simulink model "matrix_rdwr_transpose_fpga"  (R2020b)
settings: Solver=FixedStepDiscrete  StartTime=0.0  StopTime=inf  RelTol=1e-3
InitFcn:
  | %hsb_FFT_2D_init;
values from neighbouring files (symbols this model uses):
  N1 = 20    [matrix_init.m]
  N2 = 20    [matrix_init.m]
libraries: hwlogicconnlib x4, simulink x1, hdlsllib x1
settings Model: DataTypeOverride=Off  Creator=The MathWorks, Inc.  LastModifiedBy=darenlee
settings DataIOCC: LimitDataPoints=on  SaveFormat=Array  SaveOutput=off  SaveTime=off  ReturnWorkspaceOutputs=off
settings OptimizationCC: BlockReduction=off  ConditionallyExecuteInputs=off  DefaultParameterBehavior=Inlined  LifeSpan=inf
settings DebuggingCC: AlgebraicLoopMsg=error  SolverPrmCheckMsg=warning  InheritedTsInSrcMsg=none  SingleTaskRateTransMsg=error  IntegerOverflowMsg=none  ParameterPrecisionLossMsg=none  AllowSymbolicDim=off  SFUnexpectedBacktrackingDiag=warning  SFNoUnconditionalDefaultTransitionDiag=warning  SFExecutionAtInitializationDiag=none  IntegerSaturationMsg=none  ArithmeticOperatorsInVariantConditions=warning
settings HardwareCC: ProdBitPerPointer=32  ProdBitPerSizeT=32  ProdBitPerPtrDiffT=32  ProdLargestAtomicFloat=None  ProdIntDivRoundTo=Undefined  ProdEndianess=Unspecified  ProdWordSize=32  ProdHWDeviceType=ASIC/FPGA->ASIC/FPGA  TargetBitPerPointer=64  TargetBitPerSizeT=64  TargetBitPerPtrDiffT=64  TargetLongLongMode=on  TargetIntDivRoundTo=Zero  TargetEndianess=LittleEndian  TargetWordSize=64  TargetHWDeviceType=Custom Processor->MATLAB Host Computer  ProdEqTarget=off
settings ModelReferenceCC: PropagateSignalLabelsOutOfModel=off
settings SFSimCC: SimUseLocalCustomCode=off  CustomCodeUndefinedFunction=UseInterfaceOnly
settings RTWCC: RTWUseLocalCustomCode=off
settings CodeAppCC: StateflowObjectComments=on
settings GRTTargetCC: TargetLangStandard=C89/C90 (ANSI)
settings ConfigComp: CovMetricSettings=dw  CovSaveCumulativeToWorkspaceVar=on  CovSaveSingleToWorkspaceVar=on  CovExternalEMLEnable=off  CovSFcnEnable=off
settings SimscapeCC: SimscapeNormalizeSystem=off

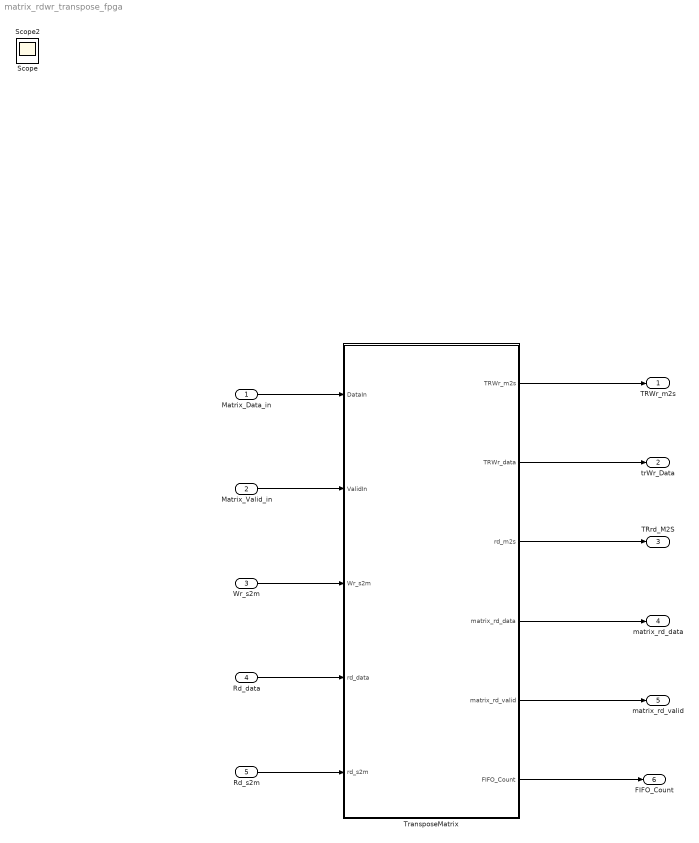
== system matrix_rdwr_transpose_fpga ==
  Matrix_Data_in : Inport  OutDataTypeStr=uint32
  Matrix_Valid_in : Inport  Port=2  OutDataTypeStr=boolean
  Wr_s2m : Inport  Port=3  OutDataTypeStr=Bus: WriteControlS2MBusObj  PortDimensions=1  BusOutputAsStruct=on
  Rd_data : Inport  Port=4  OutDataTypeStr=fixdt(0,32,0)  PortDimensions=1
  Rd_s2m : Inport  Port=5  OutDataTypeStr=Bus: ReadControlS2MBusObj  BusOutputAsStruct=on
  TransposeMatrix : Subsystem  TreatAsAtomicUnit=on
  TRWr_m2s : Outport  OutDataTypeStr=Bus: WriteControlM2SBusObj  PortDimensions=1  VectorParamsAs1DForOutWhenUnconnected=off  BusOutputAsStruct=on
  trWr_Data : Outport  Port=2  PortDimensions=1  VectorParamsAs1DForOutWhenUnconnected=off  BusOutputAsStruct=on
  TRrd_M2S : Outport  Port=3  OutDataTypeStr=Bus: ReadControlM2SBusObj  BusOutputAsStruct=on
  matrix_rd_data : Outport  Port=4
  matrix_rd_valid : Outport  Port=5
  FIFO_Count : Outport  Port=6
  Scope : Scope
  Scope2 : Scope
  wires:
  Rd_data/1 -> TransposeMatrix/4(rd_data)
  TransposeMatrix/5(matrix_rd_valid) -> matrix_rd_valid/1
  Matrix_Valid_in/1 -> TransposeMatrix/2(ValidIn)
  TransposeMatrix/4(matrix_rd_data) -> matrix_rd_data/1
  Rd_s2m/1 -> TransposeMatrix/5(rd_s2m)
  Matrix_Data_in/1 -> TransposeMatrix/1(DataIn)
  TransposeMatrix/2(TRWr_data) -> trWr_Data/1
  Wr_s2m/1 -> TransposeMatrix/3(Wr_s2m)
  TransposeMatrix/3(rd_m2s) -> TRrd_M2S/1
  TransposeMatrix/1(TRWr_m2s) -> TRWr_m2s/1
  TransposeMatrix/6(FIFO_Count) -> FIFO_Count/1

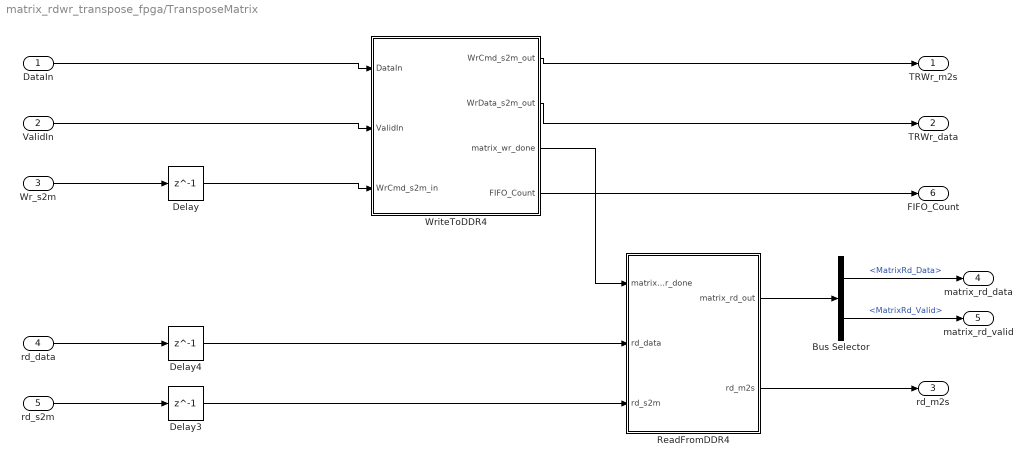
== system matrix_rdwr_transpose_fpga/TransposeMatrix ==
  DataIn : Inport
  ValidIn : Inport  Port=2
  Wr_s2m : Inport  Port=3  SampleTime=1
  rd_data : Inport  Port=4  SampleTime=1
  rd_s2m : Inport  Port=5  SampleTime=1
  Bus Selector : BusSelector  OutputSignals=MatrixRd_Data,MatrixRd_Valid
  Delay : Delay  DelayLength=1
  Delay3 : Delay  DelayLength=1
  Delay4 : Delay  DelayLength=1
  ReadFromDDR4 : Subsystem
  WriteToDDR4 : Subsystem
  TRWr_m2s : Outport  SampleTime=1  VectorParamsAs1DForOutWhenUnconnected=off
  TRWr_data : Outport  Port=2  SampleTime=1  VectorParamsAs1DForOutWhenUnconnected=off
  rd_m2s : Outport  Port=3
  matrix_rd_data : Outport  Port=4
  matrix_rd_valid : Outport  Port=5
  FIFO_Count : Outport  Port=6
  wires:
  rd_data/1 -> Delay4/1
  rd_s2m/1 -> Delay3/1
  Wr_s2m/1 -> Delay/1
  DataIn/1 -> WriteToDDR4/1(DataIn)
  ValidIn/1 -> WriteToDDR4/2(ValidIn)
  Delay/1 -> WriteToDDR4/3(WrCmd_s2m_in)
  WriteToDDR4/1(WrCmd_s2m_out) -> TRWr_m2s/1
  WriteToDDR4/2(WrData_s2m_out) -> TRWr_data/1
  Delay4/1 -> ReadFromDDR4/2(rd_data)
  Delay3/1 -> ReadFromDDR4/3(rd_s2m)
  ReadFromDDR4/2(rd_m2s) -> rd_m2s/1
  WriteToDDR4/3(matrix_wr_done) -> ReadFromDDR4/1(matrix_wr_done)
  ReadFromDDR4/1(matrix_rd_out) -> Bus Selector/1
  Bus Selector/1 -> matrix_rd_data/1  "<MatrixRd_Data>"
  Bus Selector/2 -> matrix_rd_valid/1  "<MatrixRd_Valid>"
  WriteToDDR4/4(FIFO_Count) -> FIFO_Count/1

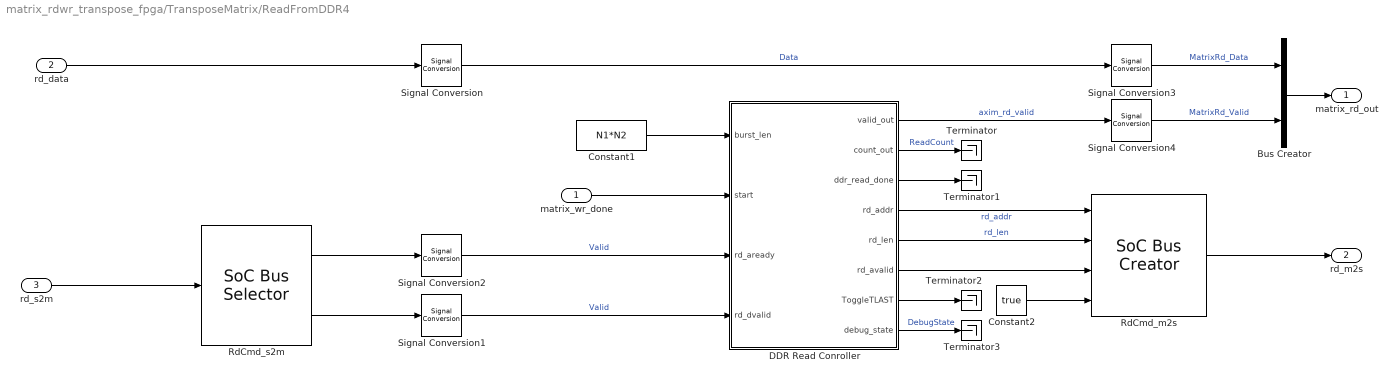
== system matrix_rdwr_transpose_fpga/TransposeMatrix/ReadFromDDR4 ==
  matrix_wr_done : Inport
  rd_data : Inport  Port=2
  rd_s2m : Inport  Port=3
  Bus Creator : BusCreator  Inputs=2
  Constant1 : Constant  Value=N1*N2  OutDataTypeStr=uint32  SampleTime=-1
  Constant2 : Constant  Value=true  SampleTime=-1
  DDR Read Conroller : MATLAB Function  TreatAsAtomicUnit=on
  RdCmd_m2s : hwlogicconnlib/SoC Bus Creator  Protocol=Random access read  ctrltype=Ready
      settings: SourceProductBaseCode=HW
  "RdCmd_s2m " : hwlogicconnlib/SoC Bus Selector  Protocol=Random access read  ctrltype=Valid
      settings: SourceProductBaseCode=HW
  Signal Conversion{,1..4} (5 alike) : SignalConversion  OverrideOpt=off
  Terminator{,1..3} (4 alike) : Terminator
  matrix_rd_out : Outport
  rd_m2s : Outport  Port=2
  wires:
  Signal Conversion1/1 -> DDR Read Conroller/4(rd_dvalid)  "Valid"
  "RdCmd_s2m "/2 -> Signal Conversion1/1
  Signal Conversion/1 -> Signal Conversion3/1  "Data"
  DDR Read Conroller/5(rd_len) -> RdCmd_m2s/2  "rd_len"
  RdCmd_m2s/1 -> rd_m2s/1
  rd_data/1 -> Signal Conversion/1
  rd_s2m/1 -> "RdCmd_s2m "/1
  matrix_wr_done/1 -> DDR Read Conroller/2(start)
  Constant1/1 -> DDR Read Conroller/1(burst_len)
  "RdCmd_s2m "/1 -> Signal Conversion2/1
  Signal Conversion2/1 -> DDR Read Conroller/3(rd_aready)  "Valid"
  DDR Read Conroller/2(count_out) -> Terminator/1  "ReadCount"
  DDR Read Conroller/1(valid_out) -> Signal Conversion4/1  "axim_rd_valid"
  DDR Read Conroller/3(ddr_read_done) -> Terminator1/1
  DDR Read Conroller/4(rd_addr) -> RdCmd_m2s/1  "rd_addr"
  DDR Read Conroller/6(rd_avalid) -> RdCmd_m2s/3
  Constant2/1 -> RdCmd_m2s/4
  DDR Read Conroller/7(ToggleTLAST) -> Terminator2/1
  DDR Read Conroller/8(debug_state) -> Terminator3/1  "DebugState"
  Signal Conversion3/1 -> Bus Creator/1  "MatrixRd_Data"
  Signal Conversion4/1 -> Bus Creator/2  "MatrixRd_Valid"
  Bus Creator/1 -> matrix_rd_out/1

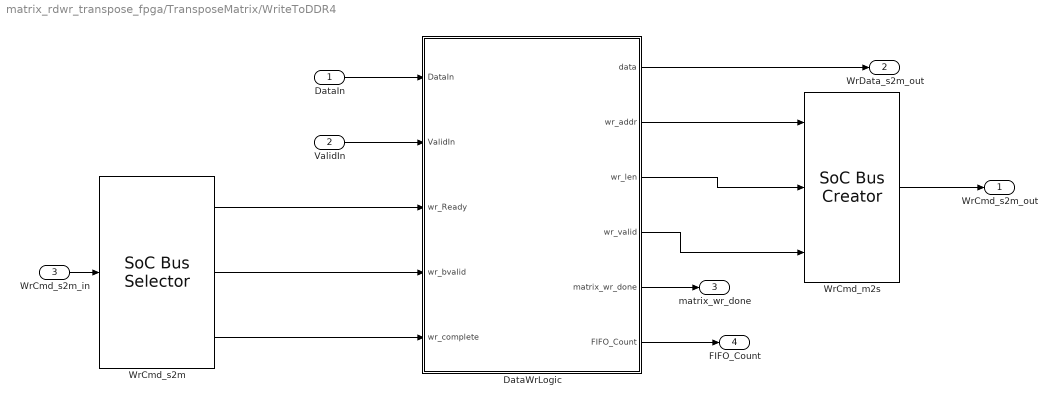
== system matrix_rdwr_transpose_fpga/TransposeMatrix/WriteToDDR4 ==
  DataIn : Inport
  ValidIn : Inport  Port=2
  WrCmd_s2m_in : Inport  Port=3
  DataWrLogic : Subsystem
  WrCmd_m2s : hwlogicconnlib/SoC Bus Creator  Protocol=Random access write  ctrltype=Valid
      settings: SourceProductBaseCode=HW
  WrCmd_s2m : hwlogicconnlib/SoC Bus Selector  Protocol=Random access write  ctrltype=Ready
      settings: SourceProductBaseCode=HW
  WrCmd_s2m_out : Outport
  WrData_s2m_out : Outport  Port=2
  matrix_wr_done : Outport  Port=3
  FIFO_Count : Outport  Port=4
  wires:
  DataWrLogic/4(wr_valid) -> WrCmd_m2s/3
  DataWrLogic/3(wr_len) -> WrCmd_m2s/2
  ValidIn/1 -> DataWrLogic/2(ValidIn)
  DataWrLogic/2(wr_addr) -> WrCmd_m2s/1
  DataWrLogic/1(data) -> WrData_s2m_out/1
  WrCmd_s2m/3 -> DataWrLogic/5(wr_complete)
  WrCmd_s2m/2 -> DataWrLogic/4(wr_bvalid)
  DataIn/1 -> DataWrLogic/1(DataIn)
  WrCmd_m2s/1 -> WrCmd_s2m_out/1
  WrCmd_s2m/1 -> DataWrLogic/3(wr_Ready)
  WrCmd_s2m_in/1 -> WrCmd_s2m/1
  DataWrLogic/5(matrix_wr_done) -> matrix_wr_done/1
  DataWrLogic/6(FIFO_Count) -> FIFO_Count/1

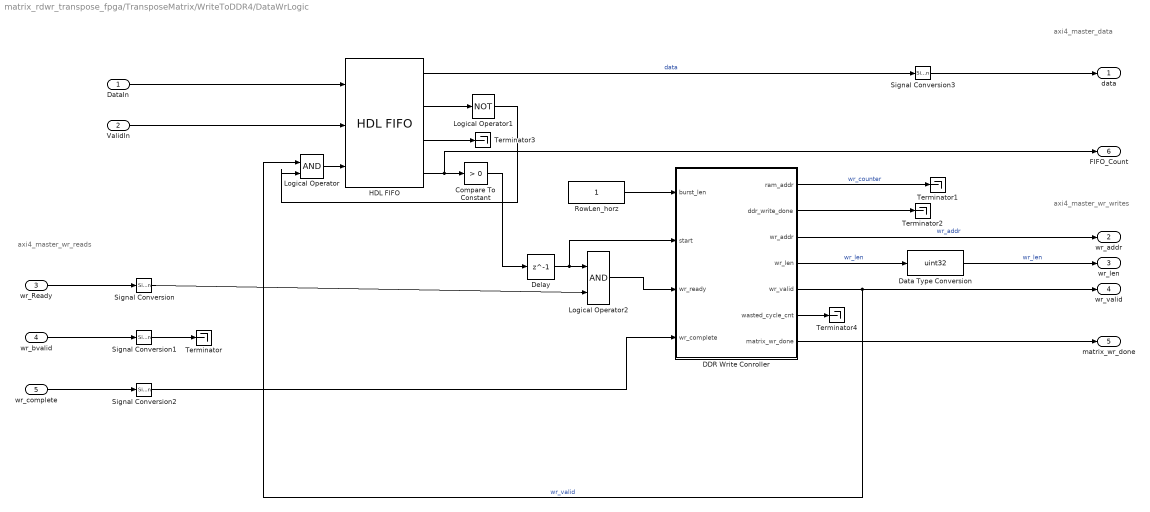
== system matrix_rdwr_transpose_fpga/TransposeMatrix/WriteToDDR4/DataWrLogic ==
  note: axi4_master_wr_reads
  note: axi4_master_wr_writes
  note: axi4_master_data
  DataIn : Inport
  ValidIn : Inport  Port=2
  wr_Ready : Inport  Port=3
  wr_bvalid : Inport  Port=4
  wr_complete : Inport  Port=5
  Compare To Constant : simulink/Logic and Bit Operations/Compare To Constant  relop=>  const=0  OutDataTypeStr=boolean
  DDR Write Conroller : MATLAB Function  TreatAsAtomicUnit=on
  Data Type Conversion : DataTypeConversion  OutDataTypeStr=uint32
  Delay : Delay  DelayLength=1
  HDL FIFO : hdlsllib/HDL RAMs/HDL FIFO  fifo_size=8192  mode=FWFT  ratio=1  push_msg=Warning  pop_msg=Warning  show_empty=on  show_full=on  show_num=on  LabelModeActiveChoice_Mode=FWFT
      settings: SourceProductBaseCode=SL
  Logical Operator : Logic  IconShape=distinctive  AllPortsSameDT=off  OutDataTypeStr=boolean
  Logical Operator1 : Logic  Operator=NOT  IconShape=distinctive  AllPortsSameDT=off  OutDataTypeStr=boolean
  Logical Operator2 : Logic  IconShape=distinctive  AllPortsSameDT=off  OutDataTypeStr=boolean
  RowLen_horz : Constant  OutDataTypeStr=uint32  SampleTime=-1
  Signal Conversion{,1..3} (4 alike) : SignalConversion  OverrideOpt=off
  Terminator{,1..4} (5 alike) : Terminator
  data : Outport
  wr_addr : Outport  Port=2
  wr_len : Outport  Port=3
  wr_valid : Outport  Port=4
  matrix_wr_done : Outport  Port=5
  FIFO_Count : Outport  Port=6
  wires:
  ValidIn/1 -> HDL FIFO/2
  DDR Write Conroller/4(wr_len) -> Data Type Conversion/1  "wr_len"
  wr_bvalid/1 -> Signal Conversion1/1
  DDR Write Conroller/3(wr_addr) -> wr_addr/1  "wr_addr"
  Data Type Conversion/1 -> wr_len/1  "wr_len"
  DataIn/1 -> HDL FIFO/1
  HDL FIFO/1 -> Signal Conversion3/1  "data"
  wr_complete/1 -> Signal Conversion2/1
  wr_Ready/1 -> Signal Conversion/1
  HDL FIFO/2 -> Logical Operator1/1
  Logical Operator/1 -> HDL FIFO/3
  Signal Conversion/1 -> Logical Operator2/2
  Logical Operator2/1 -> DDR Write Conroller/3(wr_ready)
  Logical Operator1/1 -> Logical Operator/2
  HDL FIFO/4 -> FIFO_Count/1, Compare To Constant/1
  Compare To Constant/1 -> Delay/1
  Signal Conversion2/1 -> DDR Write Conroller/4(wr_complete)
  RowLen_horz/1 -> DDR Write Conroller/1(burst_len)
  Signal Conversion1/1 -> Terminator/1
  DDR Write Conroller/5(wr_valid) -> Logical Operator/1, wr_valid/1  "wr_valid"
  DDR Write Conroller/1(ram_addr) -> Terminator1/1  "wr_counter"
  DDR Write Conroller/2(ddr_write_done) -> Terminator2/1
  Signal Conversion3/1 -> data/1
  HDL FIFO/3 -> Terminator3/1
  Delay/1 -> DDR Write Conroller/2(start), Logical Operator2/1
  DDR Write Conroller/6(wasted_cycle_cnt) -> Terminator4/1
  DDR Write Conroller/7(matrix_wr_done) -> matrix_wr_done/1

== matlab function matrix_rdwr_transpose_fpga/TransposeMatrix/WriteToDDR4/DataWrLogic/DDR Write Conroller ==
  data: ram_addr output; ddr_write_done output; burst_len input; start input boolean; wr_ready input; wr_addr output; wr_len output; wr_valid output; wr_complete input; wasted_cycle_cnt output; matrix_wr_done output; N1 parameter uint32; N2 parameter uint32
function [ram_addr, ddr_write_done, wr_addr, wr_len, wr_valid, wasted_cycle_cnt, matrix_wr_done] = ...
    hdlcoder_external_memory_write_ctrl_custom(burst_len, start, wr_ready, wr_complete, N1, N2)
%% hdlcoder_external_memory_write_ctrl_custom
%
% % State-machine behavior for writing to DDR4

%   Copyright 2017 The MathWorks, Inc.

% create persistent variables (registers)
persistent wstate burst_stop burst_count wasted_cycle_count
persistent addr_value addr_offset_add
if(isempty(wstate))
    wstate      = fi(0, 0, 4, 0);
    burst_stop  = uint32(0);
    burst_count = uint32(0);
    wasted_cycle_count = uint32(0);    
    addr_value = uint32(0);
    addr_offset_add = uint32(0);
end
wasted_cycle_cnt = cast(0,'like',wasted_cycle_count);

% state machine encoding
IDLE              = fi(0, 0, 4, 0);
WRITE_BURST_START = fi(1, 0, 4, 0);
DATA_COUNT        = fi(2, 0, 4, 0);
ACK_WAIT          = fi(3, 0, 4, 0);

DATA_BYTE_SIZE = uint32(4); % 32-bits = 4 bytes


% state machine logic
switch (wstate)
    case IDLE
        % output to AXI4 Master
        wr_addr  = uint32(0); % 4-byte address
        wr_len   = uint32(0);
        wr_valid = false;
        
        % output to DUT logic
        ram_addr = uint32(0);
        ddr_write_done = true;
        matrix_wr_done = false;
        
        % state variables
        burst_stop  = uint32(burst_len);
        burst_count = uint32(0);
        
        if start
            wstate(:) = WRITE_BURST_START;
        else
            wstate(:) = IDLE;
        end
        
        
    case WRITE_BURST_START
        % output to AXI4 Master
        wr_addr  = uint32((addr_value+addr_offset_add)*DATA_BYTE_SIZE); % convert to bytes
        wr_len   = uint32(burst_stop);
        wr_valid = false;
        
        % output to DUT logic
        ram_addr = uint32(burst_count);
        ddr_write_done = false;
        matrix_wr_done = false;    
        
        if wr_ready
            wstate(:) = DATA_COUNT;
        else
            wstate(:) = WRITE_BURST_START;
            wasted_cycle_count = uint32(wasted_cycle_count+1);
        end
        
        
    case DATA_COUNT
        % output to AXI4 Master
        wr_addr  = uint32((addr_value+addr_offset_add)*DATA_BYTE_SIZE); % convert to bytes
        wr_len   = uint32(burst_stop);
        wr_valid = true;
        
        % state variables
        burst_count = uint32(burst_count + 1);
        
        % output to DUT logic
        ram_addr = uint32(burst_count);
        ddr_write_done = false;
        matrix_wr_done = false;
        
        if ( burst_count == burst_stop )
            wstate(:) = ACK_WAIT;            
        else
            if ( wr_ready )
                wstate(:) = DATA_COUNT;
            else
                wstate(:) = WRITE_BURST_START;
            end
        end
        
        
    case ACK_WAIT
        % output to AXI4 Master
        wr_addr  = uint32(0);
        wr_len   = uint32(0);
        wr_valid = false;
        
        % output to DUT logic
        ram_addr = uint32(0);
        ddr_write_done = false;
        matrix_wr_done = false;
        
        if wr_complete
            wstate(:) = IDLE;
                   
            if addr_value < (N2*(N1-1)) % Address stride will be 0:N2:N2*(N1-1)
                % Small example (N1=4,N2=5):
                %   0 1 2 3 4
                %   5 6 7 8 9
                %   10 11... etc 
                addr_value(:) = addr_value + (N2);
            else
                
                if addr_offset_add < (N2-1)  % Will add an offset value to above addresses for each column
                                             % Using the small N1=4 and
                                             % N2=5 example...
                                             % 0,1,2,3,4 are used to offset
                                             % the above addreses
                                             % horizontally
                    addr_offset_add(:) = addr_offset_add + 1;
                else
                    addr_offset_add(:) = 0;
                    matrix_wr_done = true; 
                end    
                
                addr_value(:) = 0 ; % perform reset on address
            end
        else
            wstate(:) = ACK_WAIT;
        end
        
    otherwise
        % output to AXI4 Master
        wr_addr = uint32(0);
        wr_len = uint32(0);
        wr_valid = false;
        matrix_wr_done = false;
        
        % output to DUT logic
        ram_addr = uint32(0);
        ddr_write_done = false;
        
        wstate(:) = IDLE;
        
end
    
% For AXI4 MM Diagonstics
wasted_cycle_cnt(:) = wasted_cycle_count;

end

% LocalWords:  AXI

== matlab function matrix_rdwr_transpose_fpga/TransposeMatrix/ReadFromDDR4/DDR Read Conroller ==
  data: valid_out output; count_out output; ddr_read_done output; burst_len input; start input boolean; rd_aready input; rd_dvalid input; rd_addr output; rd_len output; rd_avalid output; ToggleTLAST output; debug_state output
function [valid_out, count_out, ddr_read_done, rd_addr, rd_len, rd_avalid,ToggleTLAST,debug_state] = ...
    hdlcoder_external_memory_read_ctrl_custom(burst_len, start, rd_aready, rd_dvalid)
%% hdlcoder_external_memory_read_ctrl_custom
%
% % State-machine behavior for reading DDR4

%   Copyright 2017 The MathWorks, Inc.

% create persistent variables (registers)
persistent rstate burst_stop burst_count
if isempty(rstate)
    rstate      = fi(0, 0, 4, 0);
    burst_stop  = uint32(0);
    burst_count = uint32(0);
    debug_state = cast(0,'like',rstate);
end

% state Memory Encoding
IDLE               = fi(0, 0, 4, 0);
READ_BURST_START   = fi(1, 0, 4, 0);
READ_BURST_REQUEST = fi(2, 0, 4, 0);
DATA_COUNT         = fi(3, 0, 4, 0);

ToggleTLAST = false;

% state machine logic
switch (rstate)
    case IDLE
        % output to AXI4 Master
        rd_addr   = uint32(0);
        rd_len    = uint32(0);
        rd_avalid = false;
        
        % output to DUT logic
        valid_out = false;
        count_out = uint32(0);
        ddr_read_done = true;
        
        % State vars
        burst_stop  = uint32(burst_len);
        burst_count = uint32(0);
        
        if start
            rstate(:) = READ_BURST_START;
        else
            rstate(:) = IDLE;
        end
        
    case READ_BURST_START
        % Daren Notes: the two pieces of information below is a read request
        %
        % rd_addr: Starting address for the read transaction that is sampled at 
        %          the first cycle of the transaction.
        % rd_len: The number of data values that you want to read, 
        %         sampled at the first cycle of the transaction.
        %
        % We only move to READ_BURST_REQUST if rd_aready is HIGH to confirm
        % DDR is ready for a readback request
        
        % output to AXI4 Master
        rd_addr   = uint32(0);  
        rd_len    = uint32(burst_stop);
        rd_avalid = false;
        
        % output to DUT logic
        valid_out = false;
        count_out = uint32(0);
        ddr_read_done = false;
        
        if rd_aready
            rstate(:) = READ_BURST_REQUEST;
        else
            rstate(:) = READ_BURST_START;
        end
        
    case READ_BURST_REQUEST
        % Daren Notes: read request
        %
        % rd_avalid: Control signal that specifies whether the read request is valid.
        %
        %
        
        % output to AXI4 Master
        rd_addr   = uint32(0);
        rd_len    = uint32(burst_stop);
        rd_avalid = true;
        
        % output to DUT logic
        valid_out = false;
        count_out = uint32(0);
        ddr_read_done = false;
        
        rstate(:) = DATA_COUNT;
        
    case DATA_COUNT
        % output to AXI4 Master
        rd_addr   = uint32(0);
        rd_len    = uint32(burst_stop);
        rd_avalid = false;
        
        % output to DUT logic
        valid_out = rd_dvalid;
        count_out = uint32(burst_count);
        ddr_read_done = false;
        
        % State vars
        if ( rd_dvalid )
            burst_count = uint32(burst_count + 1);
        end
        
        if ( burst_count == burst_stop )
            rstate(:) = IDLE;
            if rd_dvalid
                ToggleTLAST = true;
            end
        else
            rstate(:) = DATA_COUNT;
        end
        
    otherwise
        % output to AXI4 Master
        rd_addr   = uint32(0);
        rd_len    = uint32(0);
        rd_avalid = false;
        
        % output to DUT logic
        valid_out = false;
        count_out = uint32(0);
        ddr_read_done = false;
        
        rstate(:) = IDLE;
end

debug_state(:) = rstate;

end

% LocalWords:  AXI
